simulink model "RCckt"  (R2020b)
settings: Solver=VariableStepAuto  StartTime=0.0  StopTime=10.0  RelTol=1e-3
model workspace (MAT data in the model file):
  C = 10
  R = 10
settings Model: Creator=com  LastModifiedBy=com

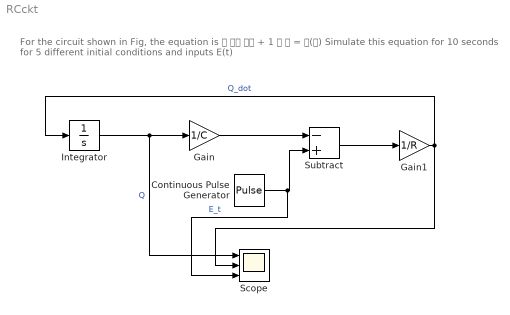
== system RCckt ==
  note: For the circuit shown in Fig, the equation is 𝑅 𝑑𝑄 𝑑𝑡 + 1 𝐶 𝑄 = 𝐸(𝑡) Simulate this equation for 10 seconds for 5 different initial conditions and inputs E(t)
  Continuous Pulse Generator : DiscretePulseGenerator  PulseType=Time based  Period=1  PulseWidth=50
  Gain : Gain  Gain=1/C
  Gain1 : Gain  Gain=1/R
  Integrator : Integrator
  Scope : Scope  NumInputPorts=3
  Subtract : Sum  Inputs=-+
  wires:
  Integrator/1 -> Scope/1, Gain/1  "Q"
  Gain/1 -> Subtract/1
  Subtract/1 -> Gain1/1
  Continuous Pulse Generator/1 -> Scope/3, Subtract/2  "E_t"
  Gain1/1 -> Integrator/1, Scope/2  "Q_dot"
